simulink model "example_quadcopter_response"  (R2016a)
settings: Solver=VariableStepAuto  StartTime=0.0  StopTime=2.5  RelTol=1e-3
settings Model: Creator=Daniel  LastModifiedBy=mgreiff
settings DataIOCC: LimitDataPoints=on
settings DebuggingCC: AllowSymbolicDim=off
settings ModelReferenceCC: PropagateSignalLabelsOutOfModel=off
settings GRTTargetCC: GeneratePreprocessorConditionals=Use local settings

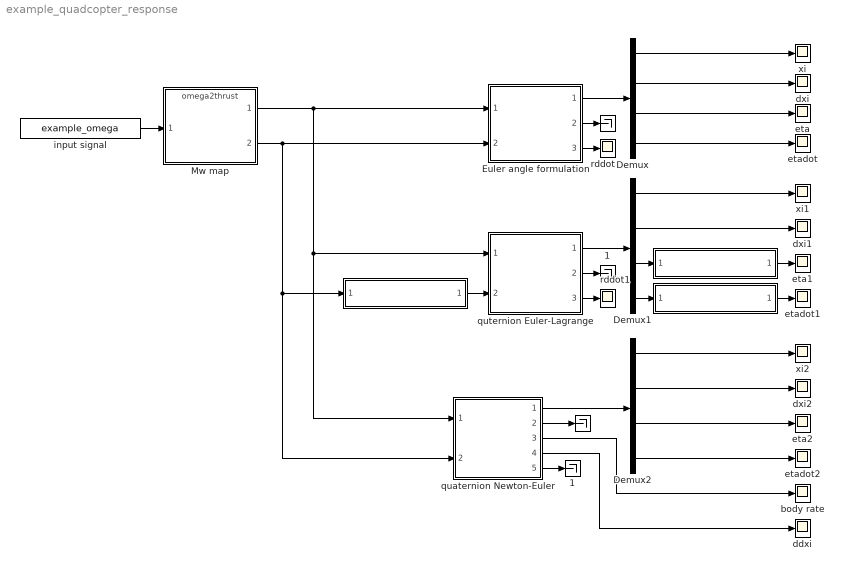
== system example_quadcopter_response ==
  " " : Terminator
  "   " : Terminator
  "    " : ModelReference  ModelNameDialog=quaternion2euler.mdl  SimulationMode=Normal  ModelReferenceVersion=1.92
  "     " : ModelReference  ModelNameDialog=quaternion2euler.mdl  SimulationMode=Normal  ModelReferenceVersion=1.92
  "          " : ModelReference  ModelNameDialog=euler2quaternion.mdl  SimulationMode=Normal  ModelReferenceVersion=1.5
  "   1" : Terminator
  " 1" : Terminator
  Demux : Demux  Outputs=[3,3,3,3]
  Demux1 : Demux  Outputs=[3,3,4,4]
  Demux2 : Demux  Outputs=[3,3,3,3]
  Euler angle formulation : ModelReference  ModelNameDialog=quadcopter_model_c_Euler.mdl  SimulationMode=Normal  ModelReferenceVersion=1.167
  Mw map : ModelReference  ModelNameDialog=omega2thrust.mdl  SimulationMode=Normal  ModelReferenceVersion=1.3
  body rate : Scope
  ddxi : Scope
  dxi : Scope
  dxi1 : Scope
  dxi2 : Scope
  eta : Scope
  eta1 : Scope
  eta2 : Scope
  etadot : Scope
  etadot1 : Scope
  etadot2 : Scope
  input signal : FromFile  FileName=example_omega  SampleTime=0.0001  ExtrapolationBeforeFirstDataPoint=Hold first value
  quaternion Newton-Euler : ModelReference  ModelNameDialog=quadcopter_model_c_NewtonEuler.mdl  SimulationMode=Normal  ModelReferenceVersion=1.320
  quternion Euler-Lagrange : ModelReference  ModelNameDialog=quadcopter_model_c_EulerLagrange.mdl  SimulationMode=Normal  ModelReferenceVersion=1.239
  rddot : Scope
  rddot1 : Scope
  xi : Scope
  xi1 : Scope
  xi2 : Scope
  wires:
  input signal/1 -> Mw map/1
  Euler angle formulation/1 -> Demux/1
  Demux/3 -> eta/1
  Demux/2 -> dxi/1
  Demux/1 -> xi/1
  Demux/4 -> etadot/1
  Mw map/2 -> quaternion Newton-Euler/2, "          "/1, Euler angle formulation/2
  Mw map/1 -> quaternion Newton-Euler/1, quternion Euler-Lagrange/1, Euler angle formulation/1
  quternion Euler-Lagrange/1 -> Demux1/1
  Demux1/3 -> "    "/1
  Demux1/2 -> dxi1/1
  Demux1/1 -> xi1/1
  "    "/1 -> eta1/1
  "          "/1 -> quternion Euler-Lagrange/2
  quaternion Newton-Euler/1 -> Demux2/1
  Demux2/2 -> dxi2/1
  Demux2/1 -> xi2/1
  Demux2/4 -> etadot2/1
  Euler angle formulation/2 -> " "/1
  Euler angle formulation/3 -> rddot/1
  Demux1/4 -> "     "/1
  "     "/1 -> etadot1/1
  Demux2/3 -> eta2/1
  quternion Euler-Lagrange/3 -> rddot1/1
  quternion Euler-Lagrange/2 -> " 1"/1
  quaternion Newton-Euler/3 -> body rate/1
  quaternion Newton-Euler/2 -> "   "/1
  quaternion Newton-Euler/4 -> ddxi/1
  quaternion Newton-Euler/5 -> "   1"/1
